simulink model "control_mimo_simulink"  (R2019b)
settings: Solver=ode45  StartTime=0.0  StopTime=500  MaxStep=0.01  RelTol=1e-3
undefined symbols (not defined in the file): A, B, C, D, xini
libraries: cstblocks x12
settings Model: Creator=B13  LastModifiedBy=l53

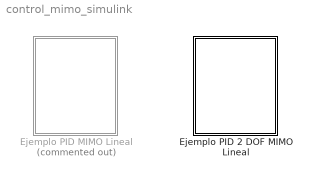
== system control_mimo_simulink ==
  Ejemplo PID 2 DOF MIMO Lineal : Subsystem
  Ejemplo PID MIMO Lineal : Subsystem  Commented=on

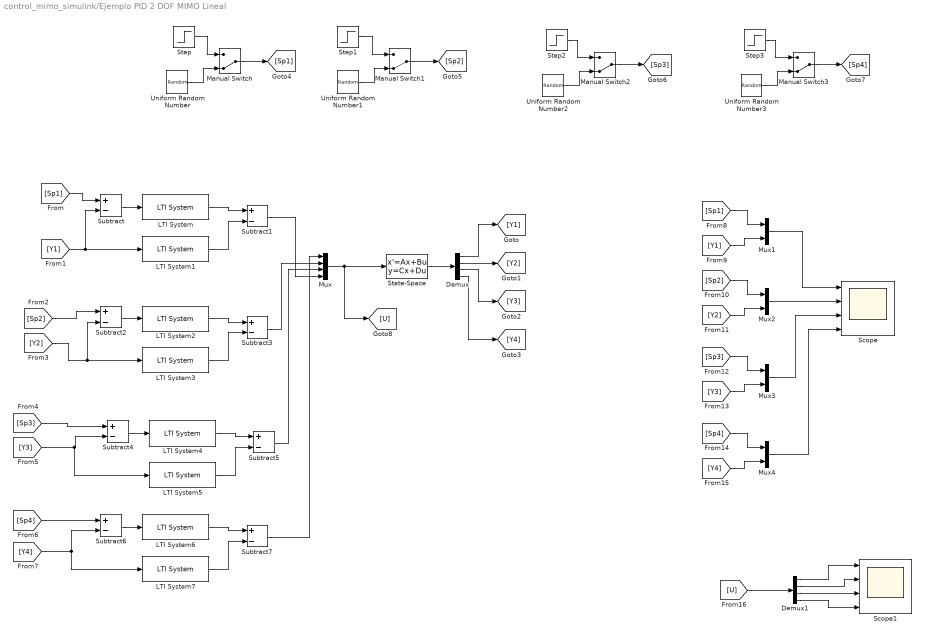
== system control_mimo_simulink/Ejemplo PID 2 DOF MIMO Lineal ==
  Demux : Demux
  Demux1 : Demux
  LTI System : cstblocks/LTI System  sys=C14a  IC=[]
  LTI System1 : cstblocks/LTI System  sys=C14b  IC=[]
  LTI System2 : cstblocks/LTI System  sys=C22a  IC=[]
  LTI System3 : cstblocks/LTI System  sys=C22b  IC=[]
  LTI System4 : cstblocks/LTI System  sys=C33a  IC=[]
  LTI System5 : cstblocks/LTI System  sys=C33b  IC=[]
  LTI System6 : cstblocks/LTI System  sys=C41a  IC=[]
  LTI System7 : cstblocks/LTI System  sys=C41b  IC=[]
  Manual Switch{,1..3} (4 alike) : ManualSwitch  CurrentSetting=0
  Mux : Mux
  Mux{1..4} (4 alike) : Mux  Inputs=2
  Scope : Scope  NumInputPorts=4
  Scope1 : Scope  NumInputPorts=4
  State-Space : StateSpace  A=A  B=B  C=C  D=D  InitialCondition=xini
  Step : Step  Time=0  After=0  SampleTime=0
  Step1 : Step  Time=0  After=0  SampleTime=0
  Step2 : Step  Time=0  After=0  SampleTime=0
  Step3 : Step  Time=0  SampleTime=0
  Subtract{,1..7} (8 alike) : Sum  Inputs=+-
  Uniform Random Number : UniformRandomNumber  SampleTime=800
  Uniform Random Number1 : UniformRandomNumber  SampleTime=1000
  Uniform Random Number2 : UniformRandomNumber  SampleTime=1200
  Uniform Random Number3 : UniformRandomNumber  SampleTime=1500
  wires:
  Mux2/1 -> Scope/2
  Step1/1 -> Manual Switch1/1
  Manual Switch/1 -> [Sp1]
  [U] -> Demux1/1
  Step2/1 -> Manual Switch2/1
  [Sp2] -> Mux2/1
  Uniform Random Number/1 -> Manual Switch/2
  [Y3] -> Mux3/2
  Demux/4 -> [Y4]
  Mux/1 -> [U], State-Space/1
  Step3/1 -> Manual Switch3/1
  Manual Switch2/1 -> [Sp3]
  Manual Switch1/1 -> [Sp2]
  Manual Switch3/1 -> [Sp4]
  Mux3/1 -> Scope/3
  Uniform Random Number2/1 -> Manual Switch2/2
  Uniform Random Number3/1 -> Manual Switch3/2
  Uniform Random Number1/1 -> Manual Switch1/2
  Step/1 -> Manual Switch/1
  Demux/2 -> [Y2]
  [Y4] -> Mux4/2
  [Sp1] -> Mux1/1
  [Sp4] -> Mux4/1
  Demux/3 -> [Y3]
  State-Space/1 -> Demux/1
  Demux/1 -> [Y1]
  Demux1/3 -> Scope1/3
  Demux1/1 -> Scope1/1
  Demux1/4 -> Scope1/4
  [Sp3] -> Mux3/1
  [Y1] -> Mux1/2
  Mux1/1 -> Scope/1
  Mux4/1 -> Scope/4
  [Y2] -> Mux2/2
  Demux1/2 -> Scope1/2
  [Sp1] -> Subtract/1
  [Y1] -> Subtract/2, LTI System1/1
  Subtract/1 -> LTI System/1
  LTI System/1 -> Subtract1/1
  LTI System1/1 -> Subtract1/2
  Subtract1/1 -> Mux/4
  [Y2] -> Subtract2/2, LTI System3/1
  [Sp2] -> Subtract2/1
  LTI System3/1 -> Subtract3/2
  LTI System2/1 -> Subtract3/1
  Subtract2/1 -> LTI System2/1
  Subtract3/1 -> Mux/2
  [Sp3] -> Subtract4/1
  LTI System5/1 -> Subtract5/2
  LTI System4/1 -> Subtract5/1
  Subtract4/1 -> LTI System4/1
  [Y3] -> LTI System5/1, Subtract4/2
  Subtract5/1 -> Mux/3
  [Sp4] -> Subtract6/1
  LTI System7/1 -> Subtract7/2
  LTI System6/1 -> Subtract7/1
  Subtract6/1 -> LTI System6/1
  [Y4] -> Subtract6/2, LTI System7/1
  Subtract7/1 -> Mux/1

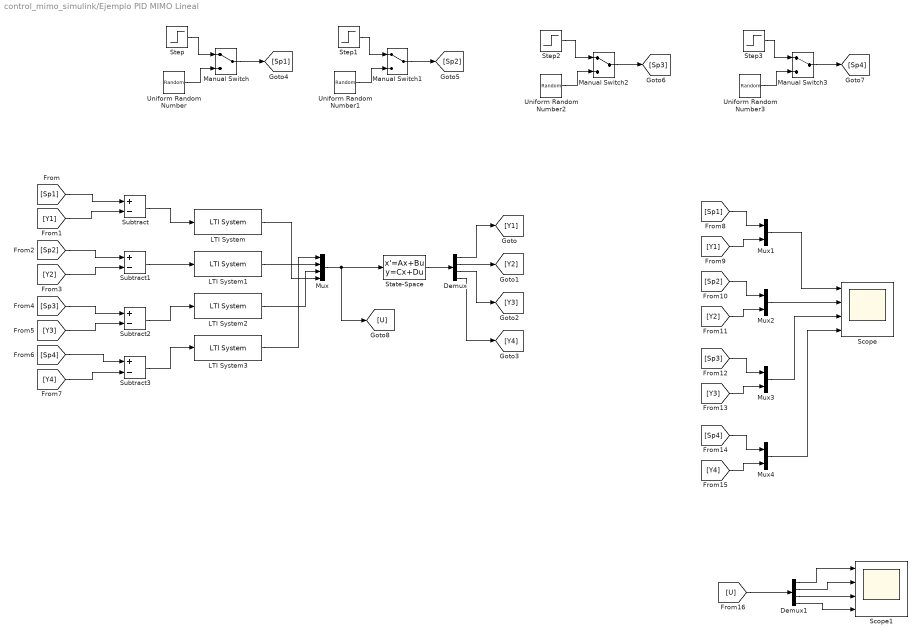
== system control_mimo_simulink/Ejemplo PID MIMO Lineal ==
  Demux : Demux
  Demux1 : Demux
  LTI System : cstblocks/LTI System  sys=C14  IC=[]
  LTI System1 : cstblocks/LTI System  sys=C22  IC=[]
  LTI System2 : cstblocks/LTI System  sys=C33  IC=[]
  LTI System3 : cstblocks/LTI System  sys=C41  IC=[]
  Manual Switch{,1..3} (4 alike) : ManualSwitch
  Mux : Mux
  Mux{1..4} (4 alike) : Mux  Inputs=2
  Scope : Scope  NumInputPorts=4
  Scope1 : Scope  NumInputPorts=4
  State-Space : StateSpace  A=A  B=B  C=C  D=D  InitialCondition=xini
  Step{,1..3} (4 alike) : Step  Time=0  After=0  SampleTime=0
  Subtract{,1..3} (4 alike) : Sum  Inputs=+-
  Uniform Random Number : UniformRandomNumber  SampleTime=500
  Uniform Random Number1 : UniformRandomNumber  SampleTime=700
  Uniform Random Number2 : UniformRandomNumber  SampleTime=900
  Uniform Random Number3 : UniformRandomNumber  SampleTime=1100
  wires:
  Mux2/1 -> Scope/2
  Step1/1 -> Manual Switch1/1
  Manual Switch/1 -> [Sp1]
  [Y1] -> Subtract/2
  [U] -> Demux1/1
  LTI System/1 -> Mux/4
  Step2/1 -> Manual Switch2/1
  [Sp2] -> Mux2/1
  Uniform Random Number/1 -> Manual Switch/2
  [Y3] -> Mux3/2
  Demux/4 -> [Y4]
  Mux/1 -> [U], State-Space/1
  Step3/1 -> Manual Switch3/1
  Subtract2/1 -> LTI System2/1
  LTI System1/1 -> Mux/2
  Manual Switch2/1 -> [Sp3]
  Manual Switch1/1 -> [Sp2]
  Subtract3/1 -> LTI System3/1
  Manual Switch3/1 -> [Sp4]
  Mux3/1 -> Scope/3
  Subtract1/1 -> LTI System1/1
  Uniform Random Number2/1 -> Manual Switch2/2
  Uniform Random Number3/1 -> Manual Switch3/2
  Uniform Random Number1/1 -> Manual Switch1/2
  Step/1 -> Manual Switch/1
  [Y3] -> Subtract2/2
  [Sp1] -> Subtract/1
  Demux/2 -> [Y2]
  [Y4] -> Mux4/2
  [Sp1] -> Mux1/1
  LTI System2/1 -> Mux/3
  [Sp4] -> Mux4/1
  [Y2] -> Subtract1/2
  [Sp2] -> Subtract1/1
  Demux/3 -> [Y3]
  [Sp3] -> Subtract2/1
  Subtract/1 -> LTI System/1
  [Sp4] -> Subtract3/1
  State-Space/1 -> Demux/1
  LTI System3/1 -> Mux/1
  [Y4] -> Subtract3/2
  Demux/1 -> [Y1]
  Demux1/3 -> Scope1/3
  Demux1/1 -> Scope1/1
  Demux1/4 -> Scope1/4
  [Sp3] -> Mux3/1
  [Y1] -> Mux1/2
  Mux1/1 -> Scope/1
  Mux4/1 -> Scope/4
  [Y2] -> Mux2/2
  Demux1/2 -> Scope1/2
